simulink model "uavQ_theta"  (R2024a)
settings: Solver=ode45  StartTime=0.0  StopTime=20  RelTol=1e-3  EnableMultiTasking=on
values from neighbouring files (symbols this model uses):
  along = [-0.0709051452518 -0.0312761201157 3.64057642679e-14 0 0 2.85492242454 -5.43216735908 -43.1077767614 0 -24.9999999995 -3.77183093786e-12 0.999999999997 ... (25 elements, 5x5)]    [data.mat]    (also in uavck_0.3ma.mat = [-0.0324066456698 -0.0020163512714 -0.000626412946339 0 -4.3)
  blong = [-8.21411807948e-14  0.0245045555074; -0.00768014371519  -4.00476593595e-05; -0.804098256542  0; 0  0; 0  0]    [data.mat]    (also in uavck_0.3ma.mat = [-0.0673606939615  3.97585187094; -0.00795176637424  -0.0012)
  clong = [1 0 0 0 0 0 57.2957795131 0 0 0 0 0 ... (25 elements, 5x5)]    [data.mat]    (also in uavck_0.3ma.mat = [0.999999999996 0 0 0 0 0 57.2957804904 0 0 0 0 0 ... (25 el)
  dlong = [0  0; 0  0; 0  0; 0  0; 0  0]    [data.mat]    (also in uavck_0.3ma.mat)
settings Model: Creator=Administrator  LastModifiedBy=rzxha
settings SolverCC: AlgebraicLoopSolver=TrustRegion
settings DataIOCC: SaveFormat=Array  SignalLoggingSaveFormat=ModelDataLogs  ReturnWorkspaceOutputs=off  SignalLoggingName=sigsOut
settings OptimizationCC: BooleanDataType=off  ExpressionDepthLimit=2147483647  InitFltsAndDblsToZero=on  LifeSpan=inf
settings DebuggingCC: SaveWithParameterizedLinksMsg=none  UnderspecifiedInitializationDetection=Classic  MergeDetectMultiDrivingBlocksExec=none  SignalResolutionControl=TryResolveAllWithWarning  MultiTaskDSMMsg=warning  MultiTaskCondExecSysMsg=none  FcnCallInpInsideContextMsg=warning  UnconnectedInputMsg=warning  UnconnectedOutputMsg=warning  UnconnectedLineMsg=warning  StateNameClashWarn=warning  SFUnexpectedBacktrackingDiag=warning  SFNoUnconditionalDefaultTransitionDiag=warning  ArithmeticOperatorsInVariantConditions=warning
settings HardwareCC: ProdBitPerPointer=32  ProdBitPerSizeT=32  ProdBitPerPtrDiffT=32  ProdLargestAtomicFloat=None  ProdIntDivRoundTo=Undefined  ProdEndianess=Unspecified  ProdWordSize=32  ProdHWDeviceType=32-bit Generic  TargetUnknown=on
settings ModelReferenceCC: EnableRefExpFcnMdlSchedulingChecks=on  PropagateSignalLabelsOutOfModel=off
settings SFSimCC: SimUseLocalCustomCode=off  CustomCodeUndefinedFunction=UseInterfaceOnly
settings RTWCC: RTWUseLocalCustomCode=off  GPUComputeCapability=3.5
settings CodeAppCC: StateflowObjectComments=on
settings GRTTargetCC: TargetFcnLib=ansi_tfl_tmw.mat  TargetLangStandard=C89/C90 (ANSI)  CombineOutputUpdateFcns=off  GRTInterface=on
settings ConfigComp: CovMetricSettings=dw  CovSaveCumulativeToWorkspaceVar=on  CovSaveSingleToWorkspaceVar=on  CovExternalEMLEnable=off

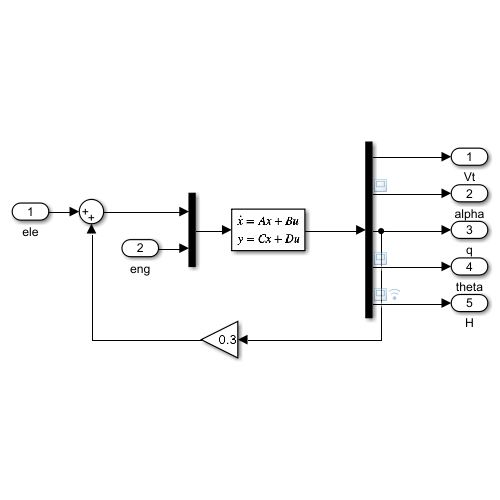
[thumbnail: Simulink's stored preview of the top-level diagram]
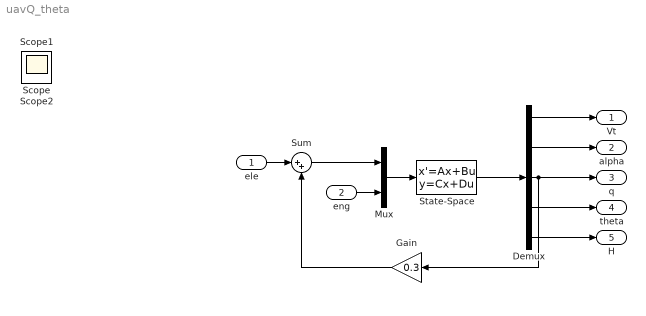
== system uavQ_theta ==
  ele : Inport
  eng : Inport  Port=2
  Demux : Demux  Outputs=5
  Gain : Gain  Gain=0.3
  Mux : Mux  Inputs=2
  State-Space : StateSpace  A=along  B=blong  C=clong  D=dlong  InitialCondition=[0 rad2deg(0) 0 rad2deg(0) 0]
  Sum : Sum  Inputs=|++
  Vt : Outport  VectorParamsAs1DForOutWhenUnconnected=off
  alpha : Outport  Port=2  VectorParamsAs1DForOutWhenUnconnected=off
  q : Outport  Port=3  VectorParamsAs1DForOutWhenUnconnected=off
  theta : Outport  Port=4  VectorParamsAs1DForOutWhenUnconnected=off
  H : Outport  Port=5  VectorParamsAs1DForOutWhenUnconnected=off
  Scope : Scope
  Scope1 : Scope
  Scope2 : Scope
  wires:
  Demux/1 -> Vt/1
  Demux/3 -> q/1, Gain/1
  Demux/4 -> theta/1
  Demux/5 -> H/1
  Demux/2 -> alpha/1
  State-Space/1 -> Demux/1
  Mux/1 -> State-Space/1
  eng/1 -> Mux/2
  Sum/1 -> Mux/1
  Gain/1 -> Sum/2
  ele/1 -> Sum/1
